simulink model "simulation_thrusters"  (R2024a)
settings: Solver=VariableStepAuto  StartTime=0.0  StopTime=10  RelTol=1e-3
values from neighbouring files (symbols this model uses):
  AUV_mass = 43.80128    [setup_auv_parameters.m]
  AUV_volume = 0.01729313024    [setup_auv_parameters.m]
  center_of_buoyancy = [0.1488 -0.74949 0.90546]    [setup_auv_parameters.m]
  center_of_gravity = [0.1488 -0.74949 0.90546]    [setup_auv_parameters.m]
  co1 = [0.04207 -0.37377 -0.14593]-center_of_gravity    [setup_auv_parameters.m]
  co2 = [0.04207 -0.37223 -0.14593]-center_of_gravity    [setup_auv_parameters.m]
  co3 = [0.04152 -0.00077 -0.34248]-center_of_gravity    [setup_auv_parameters.m]
  co4 = [0.598 0.02243 -0.02538]-center_of_gravity    [setup_auv_parameters.m]
  co5 = [-0.55567 0.02243 -0.02538]-center_of_gravity    [setup_auv_parameters.m]
  co6 = [0.04152 -0.00077 -0.35272]-center_of_gravity    [setup_auv_parameters.m]
  do1 = [0 0 1]    [setup_auv_parameters.m]
  do2 = [0 0 1]    [setup_auv_parameters.m]
  do3 = [1 0 0]    [setup_auv_parameters.m]
  do4 = [0 1 0]    [setup_auv_parameters.m]
  do5 = [0 1 0]    [setup_auv_parameters.m]
  do6 = [1 0 0]    [setup_auv_parameters.m]
  gravity_accel = 9.81    [setup_auv_parameters.m]
  water_density = 1025    [setup_auv_parameters.m]
libraries: matrix_library x8, robotcorelib x2, sim3dlib x2, shared6dof x1
settings Model: Creator=ayush  LastModifiedBy=ayush

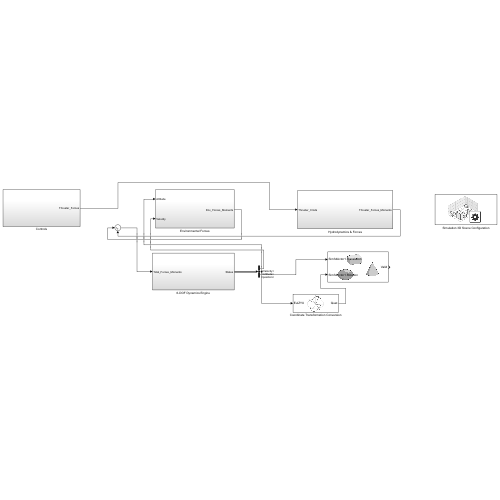
[thumbnail: Simulink's stored preview of the top-level diagram]
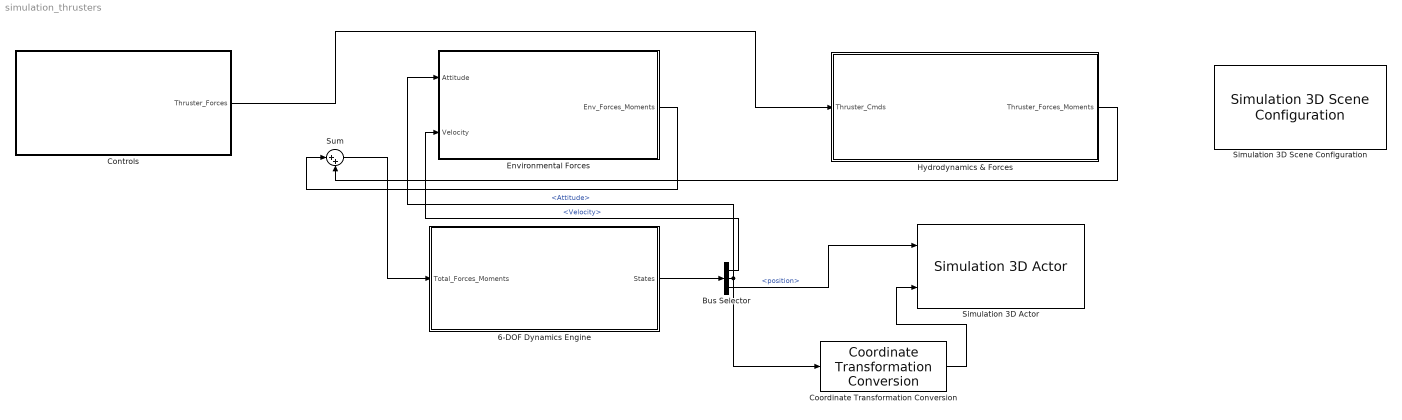
== system simulation_thrusters ==
  6-DOF Dynamics Engine : Subsystem
  Bus Selector : BusSelector  OutputSignals=Velocity,Attitude,position
  Controls : Subsystem
  Coordinate Transformation Conversion : robotcorelib/Coordinate Transformation Conversion  InputRepresentation=Euler Angles  InputEulerSequence=ZYX  ShowTrVecInputPort=on  OutputRepresentation=Quaternion  OutputEulerSequence=ZYX  ShowTrVecOutputPort=on  SimulateUsing=Interpreted execution
      settings: LibrarySourceBlock=uavutilslib/Coordinate Transformation Conversion
  Environmental Forces : Subsystem
  Hydrodynamics & Forces : Subsystem
  Simulation 3D Actor : sim3dlib/Simulation 3D Actor  Priority=1  ActorName=BP_AUV  ParentName=Scene Origin  Operation=Reference by name  InitScriptText=|  SampleTime=-1  Translation=single([0 0 0])  Rotation=single([0 0 0])  Scale=single([1 1 1])  InputsText=Sim3dActor1.Translation Sim3dActor1.Rotation  aMode=5  ActorTag=Sim3dActor1  ActorType=Sim3dActor  ID=1
      | % Reserved keywords:
      | % - Actor : handle to this actor object
      | % - World : handle to the world object
      | 
      | % Examples:
      | 
      | % Create a primitive geometry (optional)
      | % Actor.createShape('box', [1 1 1]);
      | 
      | % Initialize values (optional)
      | % Actor.Scale = 1;
      | % Actor.Color = [1 0 0];
  Simulation 3D Scene Configuration : sim3dlib/Simulation 3D Scene Configuration  Priority=0  ProjectFormat=Unreal Editor  SceneDesc=US city block  ProjectName=C:\Program Files\MATLAB\R2024a\toolbox\shared\sim3d_projects\automotive_project_windows\UE\WindowsNoEditor\VehicleSimulation.exe  ScenePath=/Game/Maps/USCityBlock  UEProjPath=D:\MyProject\MyProject.uproject  EnableOpenDRIVE=off  vehTagList={'Custom';'Scene Origin'}  vehTag=Scene Origin  FreeCameraInitialTranslation=[0, 0, 0]  FreeCameraDefaultInitialTranslation=[-6, 0, 2]  FreeCameraInitialRotation=[0, 0, 0]  FreeCameraDefaultInitialRotation=[0, -15, 0]  OpVisEn=off  Ts=1/60  EnableWindow=on  EnableRemoteAccess=off  EnableWeather=off  SunAzimuth=90  SunAltitude=40.0  EnableGeospatialSun=off  Latitude=0  Longitude=0  Date=2023-01-01  Time=10:30:00  GeoTimeZone=-5.0  SunDaylightSaving=off  wind=1  clouds=10  EnableVolumetricClouds=off  CloudCoverage=0  CloudAltitude=6  fog=0  rain=0  RaindropsEffect=off  SnowDensity=0  EnableGeospatial=off  UseTrueOrigin=off  OriginHeight=200  OriginLatitude=40.744652  OriginLongitude=-73.988864  MapStyle=Aerial  AdditionalAssetIDs=[]  UseAdvancedSunSky=off  SolarTime=11  TimeZone=-5  Day=21  Month=9  Year=2022  UseDaylightSavingTime=on  DSTStartDay=10  DSTStartMonth=3  DSTEndDay=3  DSTEndMonth=11  DSTSwitchHour=2  sensorTag=MainCamera1  sensorId=1  sensorName=MainCamera1  mountLoc=Origin  offsetFlag=off  tmountOffset=[0, 0, 0]  rmountOffset=[0, 0, 0]  HorizontalResolution=1280  VerticalResolution=720  HorizontalFOV=60  mountPoint=[0 0 0]  mountOrientation=[0 0 0]  aMode=4  ID=1  GeoTrigger=Inactive
      settings: LibrarySourceBlock=uavsim3dlib/Simulation 3D Scene Configuration
  Sum : Sum  Inputs=|++
  wires:
  Environmental Forces/1(Env_Forces_Moments) -> Sum/1
  Hydrodynamics & Forces/1(Thruster_Forces_Moments) -> Sum/2
  Sum/1 -> 6-DOF Dynamics Engine/1(Total_Forces_Moments)
  6-DOF Dynamics Engine/1(States) -> Bus Selector/1
  Controls/1(Thruster_Forces) -> Hydrodynamics & Forces/1(Thruster_Cmds)
  Bus Selector/2 -> Coordinate Transformation Conversion/1, Environmental Forces/1(Attitude)  "<Attitude>"
  Bus Selector/1 -> Environmental Forces/2(Velocity)  "<Velocity>"
  Bus Selector/3 -> Simulation 3D Actor/1  "<position>"
  Coordinate Transformation Conversion/1 -> Simulation 3D Actor/2

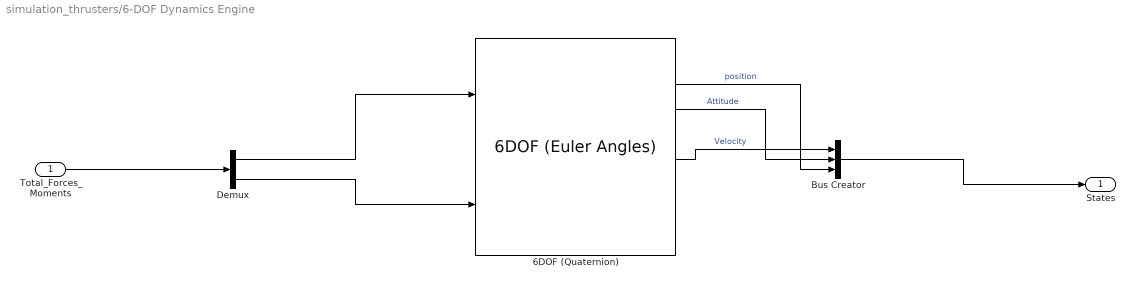
== system simulation_thrusters/6-DOF Dynamics Engine ==
  Total_Forces_Moments : Inport
  6DOF (Quaternion) : shared6dof/6DOF (Euler Angles)  units=Metric (MKS)  mtype=Fixed  rep=Quaternion  xme_0=[0 0 0]  Vm_0=[0 0 0]  eul_0=[0 0 0]  pm_0=[0 0 0]  mass_0=1.0  mass_e=0.5  mass_f=2.0  inertia=eye(3)  inertia_e=eye(3)  inertia_f=2*eye(3)  k_quat=1.0  vre_flag=on  abi_flag=off  aMode=0  xme_statename=''  Vm_statename=''  eul_statename=''  quat_statename=''  pm_statename=''  mass_statename=''
      settings: LibrarySourceBlock=aerolib6dof2/6DOF (Quaternion)
  Bus Creator : BusCreator  Inputs=3
  Demux : Demux  Outputs=2
  States : Outport
  wires:
  Bus Creator/1 -> States/1
  6DOF (Quaternion)/5 -> Bus Creator/1  "Velocity"
  6DOF (Quaternion)/3 -> Bus Creator/2  "Attitude"
  Total_Forces_Moments/1 -> Demux/1
  Demux/1 -> 6DOF (Quaternion)/1
  Demux/2 -> 6DOF (Quaternion)/2
  6DOF (Quaternion)/2 -> Bus Creator/3  "position"

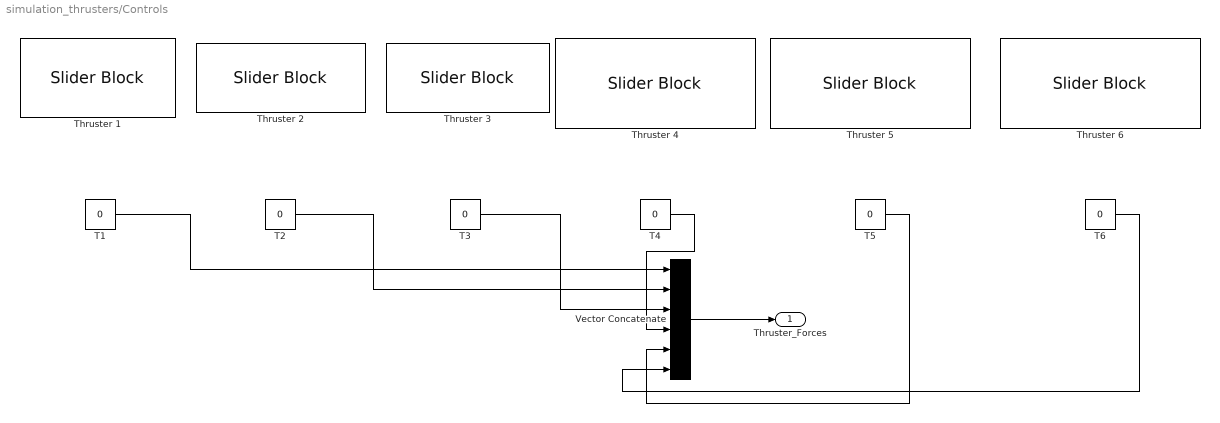
== system simulation_thrusters/Controls ==
  T{1..6} (6 alike) : Constant  Value=0
  Thruster 1 : SliderBlock  LabelPosition=Hide
  Thruster {2..6} (5 alike) : SliderBlock
  Vector Concatenate : Concatenate  NumInputs=6
  Thruster_Forces : Outport
  wires:
  T1/1 -> Vector Concatenate/1
  T2/1 -> Vector Concatenate/2
  T3/1 -> Vector Concatenate/3
  T4/1 -> Vector Concatenate/4
  T5/1 -> Vector Concatenate/5
  T6/1 -> Vector Concatenate/6
  Vector Concatenate/1 -> Thruster_Forces/1

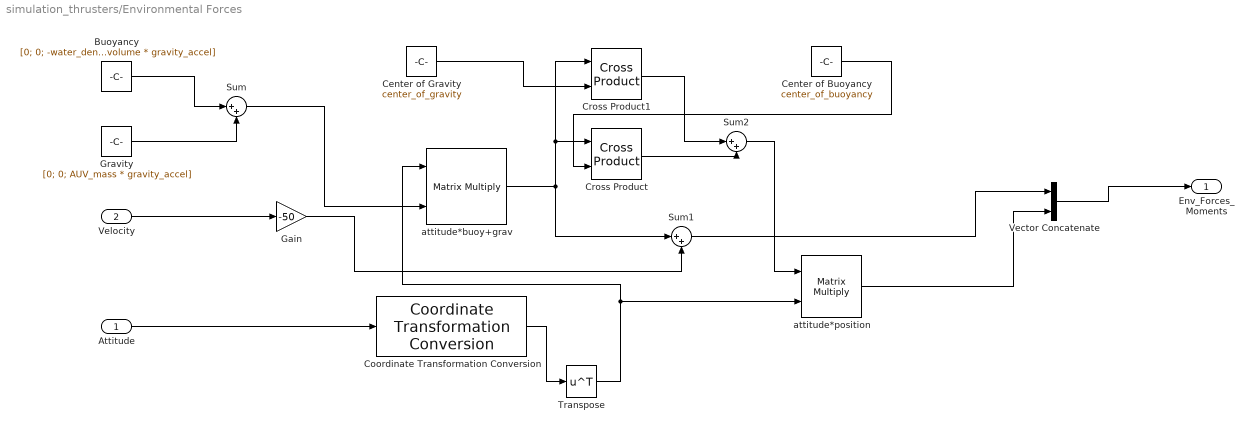
== system simulation_thrusters/Environmental Forces ==
  Attitude : Inport
  Velocity : Inport  Port=2
  Buoyancy : Constant  Value=[0; 0; -water_density * AUV_volume * gravity_accel]
  Center of Buoyancy : Constant  Value=center_of_buoyancy
  Center of Gravity : Constant  Value=center_of_gravity
  Coordinate Transformation Conversion : robotcorelib/Coordinate Transformation Conversion  InputRepresentation=Euler Angles  InputEulerSequence=ZYX  ShowTrVecInputPort=on  OutputRepresentation=Rotation Matrix  OutputEulerSequence=ZYX  ShowTrVecOutputPort=on  SimulateUsing=Interpreted execution
      settings: LibrarySourceBlock=navlib/Utilities/Coordinate Transformation Conversion
  Cross Product : matrix_library/Cross Product
  Cross Product1 : matrix_library/Cross Product
  Gain : Gain  Gain=-50
  Gravity : Constant  Value=[0; 0; AUV_mass * gravity_accel]
  Sum : Sum  Inputs=|++
  Sum1 : Sum  Inputs=|++
  Sum2 : Sum  Inputs=|++
  Transpose : Math  Operator=transpose
  Vector Concatenate : Concatenate
  attitude*buoy+grav : Product  Multiplication=Matrix(*)
  attitude*position : Product  Multiplication=Matrix(*)
  Env_Forces_Moments : Outport
  wires:
  Velocity/1 -> Gain/1
  Attitude/1 -> Coordinate Transformation Conversion/1
  Coordinate Transformation Conversion/1 -> Transpose/1
  Transpose/1 -> attitude*position/2, attitude*buoy+grav/1
  Buoyancy/1 -> Sum/1
  Gravity/1 -> Sum/2
  Sum/1 -> attitude*buoy+grav/2
  Gain/1 -> Sum1/2
  attitude*buoy+grav/1 -> Cross Product1/1, Cross Product/1, Sum1/1
  Cross Product1/1 -> Sum2/1
  Cross Product/1 -> Sum2/2
  Sum1/1 -> Vector Concatenate/1
  Vector Concatenate/1 -> Env_Forces_Moments/1
  Sum2/1 -> attitude*position/1
  attitude*position/1 -> Vector Concatenate/2
  Center of Gravity/1 -> Cross Product1/2
  Center of Buoyancy/1 -> Cross Product/2

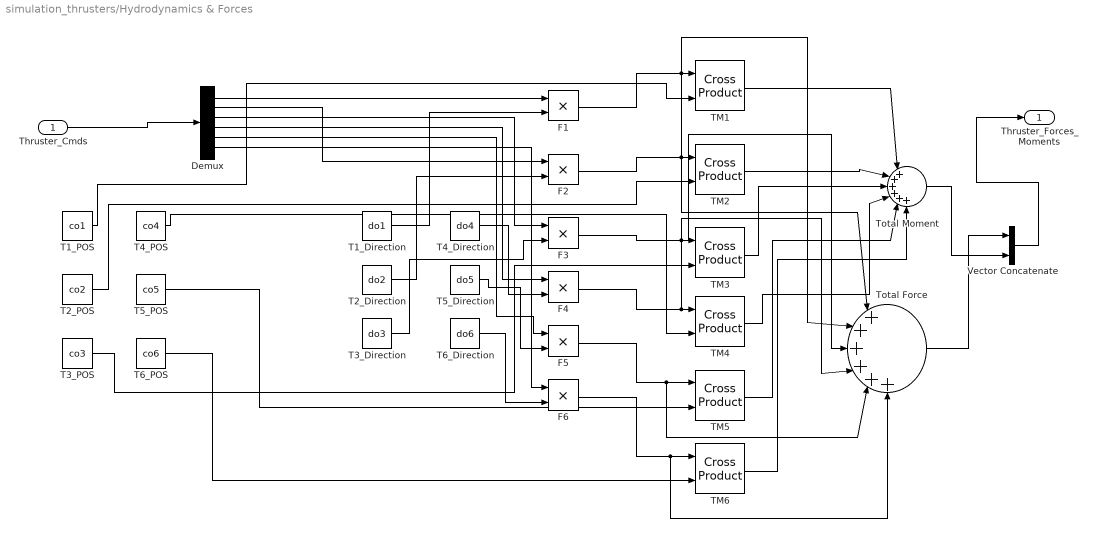
== system simulation_thrusters/Hydrodynamics & Forces ==
  Thruster_Cmds : Inport
  Demux : Demux  Outputs=6
  F{1..6} (6 alike) : Product
  T1_Direction : Constant  Value=do1
  T1_POS : Constant  Value=co1
  T2_Direction : Constant  Value=do2
  T2_POS : Constant  Value=co2
  T3_Direction : Constant  Value=do3
  T3_POS : Constant  Value=co3
  T4_Direction : Constant  Value=do4
  T4_POS : Constant  Value=co4
  T5_Direction : Constant  Value=do5
  T5_POS : Constant  Value=co5
  T6_Direction : Constant  Value=do6
  T6_POS : Constant  Value=co6
  TM{1..6} (6 alike) : matrix_library/Cross Product
  Total Force : Sum  Inputs=|++++++
  Total Moment : Sum  Inputs=|++++++
  Vector Concatenate : Concatenate
  Thruster_Forces_Moments : Outport
  wires:
  Thruster_Cmds/1 -> Demux/1
  Demux/1 -> F1/1
  T1_Direction/1 -> F1/2
  T2_Direction/1 -> F2/2
  Demux/2 -> F2/1
  Demux/3 -> F3/1
  Demux/4 -> F4/1
  Demux/5 -> F5/1
  Demux/6 -> F6/1
  T3_Direction/1 -> F3/2
  T4_Direction/1 -> F4/2
  T5_Direction/1 -> F5/2
  T6_Direction/1 -> F6/2
  F1/1 -> Total Force/1, TM1/1
  F2/1 -> Total Force/2, TM2/1
  F3/1 -> Total Force/3, TM3/1
  F4/1 -> Total Force/4, TM4/1
  F5/1 -> TM5/1, Total Force/5
  F6/1 -> TM6/1, Total Force/6
  T1_POS/1 -> TM1/2
  T2_POS/1 -> TM2/2
  T3_POS/1 -> TM3/2
  T4_POS/1 -> TM4/2
  T5_POS/1 -> TM5/2
  T6_POS/1 -> TM6/2
  TM1/1 -> Total Moment/1
  TM2/1 -> Total Moment/2
  TM3/1 -> Total Moment/3
  TM4/1 -> Total Moment/4
  TM5/1 -> Total Moment/5
  TM6/1 -> Total Moment/6
  Total Force/1 -> Vector Concatenate/1
  Total Moment/1 -> Vector Concatenate/2
  Vector Concatenate/1 -> Thruster_Forces_Moments/1
